simulink model "nonlinear_model"  (R2016b)
settings: Solver=VariableStepAuto  StartTime=0.0  StopTime=30  RelTol=1e-3
values from neighbouring files (symbols this model uses):
  j_e = m_c*(l_c)^2 + 2*m_p*(l_h)^2    (= 1.033536)    [P3p2_init.m]    (also in init_heli_all.m)
  j_lambda = m_c*(l_c)^2 + 2*m_p*((l_h)^2 + (l_p)^2)    (= 1.077636)    [P3p2_init.m]    (also in init_heli_all.m)
  j_p = 2*m_p*(l_p)^2    (= 0.0441)    [P3p2_init.m]    (also in init_heli_all.m)
  K = lqr(A, B, Q, R)    [P3p2_init.m]    (also in init_heli_all.m)
  L1 = l_h*k_f    (= 0.10164)    [init_heli_all.m]
  L2 = k2*j_e    (= 0.10164)    [init_heli_all.m]
  L3 = l_h*k_f    (= 0.10164)    [init_heli_all.m]
  L4 = k_f*l_h*l_p    (= 0.017787)    [init_heli_all.m]
  P = inv(C*inv(B*K-A)*B)    [P3p2_init.m]    (also in init_heli_all.m)
settings Model: Creator=Kevin K. Kaldvansvik  LastModifiedBy=Kevin K. Kaldvansvik

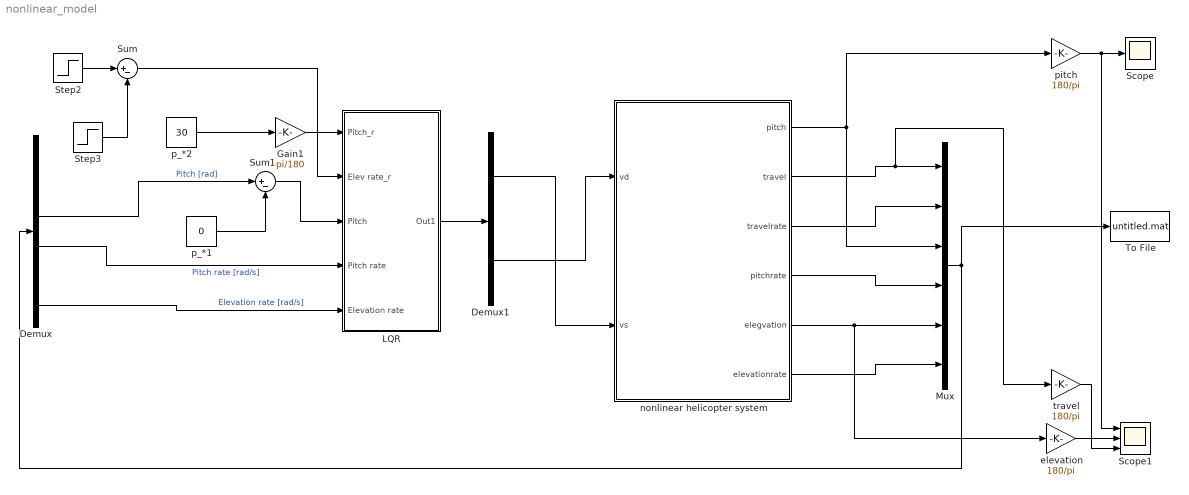
== system nonlinear_model ==
  Demux : Demux  Outputs=6
  Demux1 : Demux  Outputs=2
  Gain1 : Gain  Gain=pi/180
  LQR : Subsystem
  Mux : Mux  Inputs=6
  Scope : Scope
  Scope1 : Scope  NumInputPorts=3
  Step2 : Step  After=pi/36  SampleTime=0
  Step3 : Step  Time=2  After=pi/36  SampleTime=0
  Sum : Sum  Inputs=|+-
  Sum1 : Sum  Inputs=|+-
  To File : ToFile  MatrixName=kp_v1
  elevation : Gain  Gain=180/pi
  nonlinear helicopter system : Subsystem
  p_*1 : Constant  Value=0
  p_*2 : Constant  Value=30
  pitch : Gain  Gain=180/pi
  "travel " : Gain  Gain=180/pi
  wires:
  p_*1/1 -> Sum1/2
  Sum1/1 -> LQR/3(Pitch)
  Demux/4 -> LQR/4(Pitch rate)  "Pitch rate [rad/s]"
  Mux/1 -> To File/1, Demux/1
  Demux/3 -> Sum1/1  "Pitch [rad]"
  pitch/1 -> Scope1/1, Scope/1
  p_*2/1 -> Gain1/1
  Gain1/1 -> LQR/1(Pitch_r)
  nonlinear helicopter system/5(elegvation) -> Mux/5, elevation/1
  nonlinear helicopter system/1(pitch) -> Mux/3, pitch/1
  nonlinear helicopter system/2(travel) -> "travel "/1, Mux/1
  nonlinear helicopter system/3(travelrate) -> Mux/2
  nonlinear helicopter system/4(pitchrate) -> Mux/4
  nonlinear helicopter system/6(elevationrate) -> Mux/6
  LQR/1(Out1) -> Demux1/1
  Demux/6 -> LQR/5(Elevation rate)  "Elevation rate [rad/s]"
  Step2/1 -> Sum/1
  Step3/1 -> Sum/2
  Sum/1 -> LQR/2(Elev rate_r)
  Demux1/1 -> nonlinear helicopter system/2(vs)
  Demux1/2 -> nonlinear helicopter system/1(vd)
  elevation/1 -> Scope1/2
  "travel "/1 -> Scope1/3

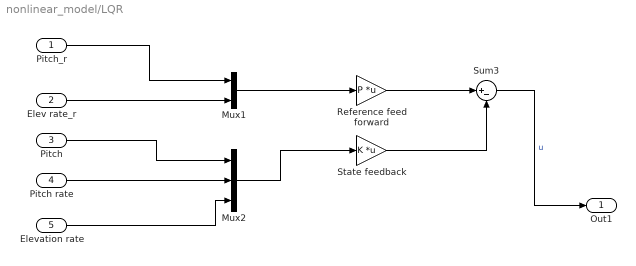
== system nonlinear_model/LQR ==
  Pitch_r : Inport
  Elev rate_r : Inport  Port=2
  Pitch : Inport  Port=3
  Pitch rate : Inport  Port=4
  Elevation rate : Inport  Port=5
  Mux1 : Mux  Inputs=2
  Mux2 : Mux  Inputs=3
  "Reference feed forward " : Gain  Gain=P  Multiplication=Matrix(K*u)
  State feedback : Gain  Gain=K  Multiplication=Matrix(K*u)
  Sum3 : Sum  Inputs=|+-
  Out1 : Outport
  wires:
  State feedback/1 -> Sum3/2
  "Reference feed forward "/1 -> Sum3/1
  Pitch/1 -> Mux2/1
  Elevation rate/1 -> Mux2/3
  Mux2/1 -> State feedback/1
  Pitch rate/1 -> Mux2/2
  Mux1/1 -> "Reference feed forward "/1
  Sum3/1 -> Out1/1  "u"
  Elev rate_r/1 -> Mux1/2
  Pitch_r/1 -> Mux1/1

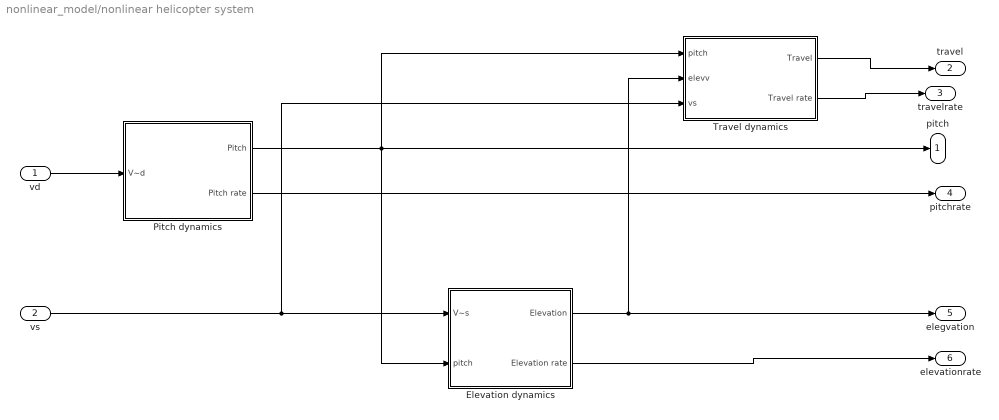
== system nonlinear_model/nonlinear helicopter system ==
  vd : Inport
  vs : Inport  Port=2
  Elevation dynamics : Subsystem
  Pitch dynamics : Subsystem
  Travel dynamics : Subsystem
  pitch : Outport
  travel : Outport  Port=2
  travelrate : Outport  Port=3
  pitchrate : Outport  Port=4
  elegvation : Outport  Port=5
  elevationrate : Outport  Port=6
  wires:
  vd/1 -> Pitch dynamics/1(V~d)
  Elevation dynamics/1(Elevation) -> Travel dynamics/2(elevv), elegvation/1
  Pitch dynamics/2(Pitch rate) -> pitchrate/1
  vs/1 -> Elevation dynamics/1(V~s), Travel dynamics/3(vs)
  Pitch dynamics/1(Pitch) -> Elevation dynamics/2(pitch), Travel dynamics/1(pitch), pitch/1
  Travel dynamics/2(Travel rate) -> travelrate/1
  Travel dynamics/1(Travel) -> travel/1
  Elevation dynamics/2(Elevation rate) -> elevationrate/1

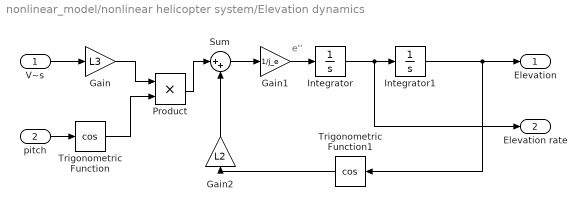
== system nonlinear_model/nonlinear helicopter system/Elevation dynamics ==
  note: e''
  V~s : Inport
  pitch : Inport  Port=2
  Gain : Gain  Gain=L3
  Gain1 : Gain  Gain=1/j_e
  Gain2 : Gain  Gain=L2
  Integrator : Integrator
  Integrator1 : Integrator
  Product : Product
  Sum : Sum  Inputs=|++
  Trigonometric Function : Trigonometry  Operator=cos
  Trigonometric Function1 : Trigonometry  Operator=cos
  Elevation : Outport
  Elevation rate : Outport  Port=2
  wires:
  Integrator/1 -> Elevation rate/1, Integrator1/1
  V~s/1 -> Gain/1
  Integrator1/1 -> Trigonometric Function1/1, Elevation/1
  Gain/1 -> Product/1
  Sum/1 -> Gain1/1
  Gain1/1 -> Integrator/1
  Product/1 -> Sum/1
  pitch/1 -> Trigonometric Function/1
  Trigonometric Function/1 -> Product/2
  Trigonometric Function1/1 -> Gain2/1
  Gain2/1 -> Sum/2

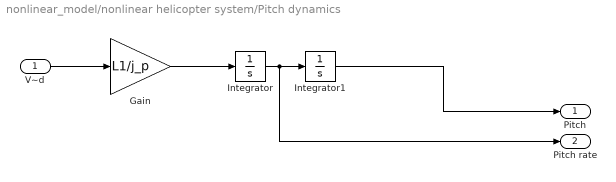
== system nonlinear_model/nonlinear helicopter system/Pitch dynamics ==
  V~d : Inport
  Gain : Gain  Gain=L1/j_p
  Integrator : Integrator
  Integrator1 : Integrator
  Pitch : Outport
  Pitch rate : Outport  Port=2
  wires:
  Integrator/1 -> Pitch rate/1, Integrator1/1
  Integrator1/1 -> Pitch/1
  V~d/1 -> Gain/1
  Gain/1 -> Integrator/1

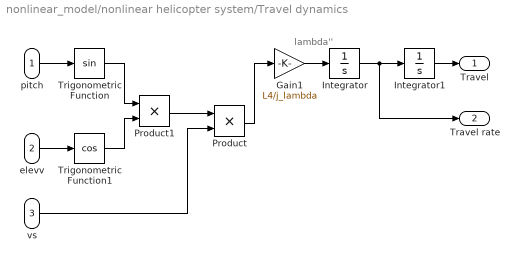
== system nonlinear_model/nonlinear helicopter system/Travel dynamics ==
  note: lambda''
  pitch : Inport
  elevv : Inport  Port=2
  vs : Inport  Port=3
  Gain1 : Gain  Gain=L4/j_lambda
  Integrator : Integrator
  Integrator1 : Integrator
  Product : Product
  Product1 : Product
  Trigonometric Function : Trigonometry
  Trigonometric Function1 : Trigonometry  Operator=cos
  Travel : Outport
  Travel rate : Outport  Port=2
  wires:
  Integrator1/1 -> Travel/1
  Integrator/1 -> Integrator1/1, Travel rate/1
  pitch/1 -> Trigonometric Function/1
  Gain1/1 -> Integrator/1
  elevv/1 -> Trigonometric Function1/1
  Product/1 -> Gain1/1
  Trigonometric Function/1 -> Product1/1
  Trigonometric Function1/1 -> Product1/2
  vs/1 -> Product/2
  Product1/1 -> Product/1
